simulink library "Lib_Turbo_Splitter_TMATS"  (R2012b)
settings: Solver=ode45  StartTime=0.0  StopTime=10.0  RelTol=1e-3
Description:
  | Thomas Modules
settings Model: Creator=jwchapm2  LastModifiedBy=jwchapm2

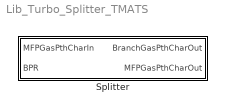
== system Lib_Turbo_Splitter_TMATS ==
  Splitter : Subsystem  mask(T-MATS: Splitter Library Block){}
      mask help: This block simulates the performance of a splitter/branch using basic flow relationships.
      mask Help: web(which('Turbo_TMATS_Splt.html'),'-helpbrowser')

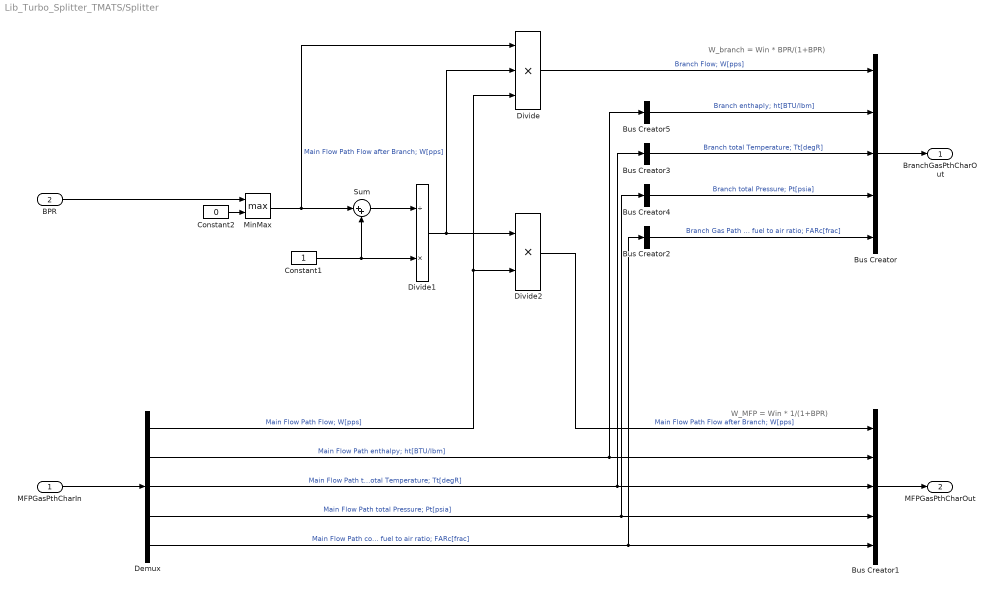
== system Lib_Turbo_Splitter_TMATS/Splitter ==
  note: W_branch = Win * BPR/(1+BPR)
  note: W_MFP = Win * 1/(1+BPR)
  MFPGasPthCharIn : Inport
  BPR : Inport  Port=2
  Bus Creator : BusCreator  Inputs=5
  Bus Creator1 : BusCreator  Inputs=5
  Bus Creator{2..5} (4 alike) : BusCreator  Inputs=1
  Constant1 : Constant
  Constant2 : Constant  Value=0
  Demux : Demux  Outputs=5
  Divide : Product  Inputs=***
  Divide1 : Product  Inputs=/*
  Divide2 : Product  Inputs=**
  MinMax : MinMax  Function=max  Inputs=2
  Sum : Sum  Inputs=|++
  BranchGasPthCharOut : Outport
  MFPGasPthCharOut : Outport  Port=2
  wires:
  Bus Creator/1 -> BranchGasPthCharOut/1
  Demux/4 -> Bus Creator4/1, Bus Creator1/4  "Main Flow Path total Pressure; Pt[psia]"
  Demux/3 -> Bus Creator3/1, Bus Creator1/3  "Main Flow Path total Temperature; Tt[degR]"
  Demux/5 -> Bus Creator2/1, Bus Creator1/5  "Main Flow Path combusted fuel to air ratio; FARc[frac]"
  MFPGasPthCharIn/1 -> Demux/1
  Bus Creator1/1 -> MFPGasPthCharOut/1
  Constant1/1 -> Sum/2, Divide1/2
  Divide2/1 -> Bus Creator1/1  "Main Flow Path Flow after Branch; W[pps]"
  Divide/1 -> Bus Creator/1  "Branch Flow; W[pps]"
  Bus Creator2/1 -> Bus Creator/5  "Branch Gas Path combusted fuel to air ratio; FARc[frac]"
  Bus Creator3/1 -> Bus Creator/3  "Branch total Temperature; Tt[degR]"
  Bus Creator4/1 -> Bus Creator/4  "Branch total Pressure; Pt[psia]"
  Sum/1 -> Divide1/1
  Demux/1 -> Divide/3, Divide2/2  "Main Flow Path Flow; W[pps]"
  Divide1/1 -> Divide/2, Divide2/1  "Main Flow Path Flow after Branch; W[pps]"
  Demux/2 -> Bus Creator5/1, Bus Creator1/2  "Main Flow Path enthalpy; ht[BTU/lbm]"
  Bus Creator5/1 -> Bus Creator/2  "Branch enthaply; ht[BTU/lbm]"
  MinMax/1 -> Divide/1, Sum/1
  Constant2/1 -> MinMax/2
  BPR/1 -> MinMax/1
